simulink subsystem "phase_interpolator"  (R2022b)
settings: Solver=VariableStepAuto  StartTime=0.0  StopTime=10.0  RelTol=1e-3
undefined symbols (not defined in the file): serial_frequency, time_precision
libraries: msbPllFoundation x1, msbUtilities x1
settings Model: Creator=Ali-Laptop  LastModifiedBy=Ali-Laptop

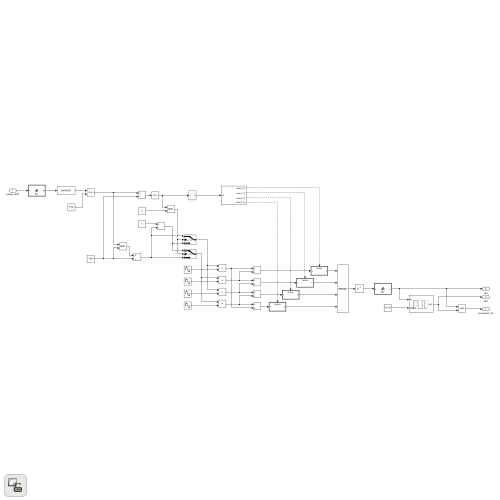
[thumbnail: Simulink's stored preview of the top-level diagram]
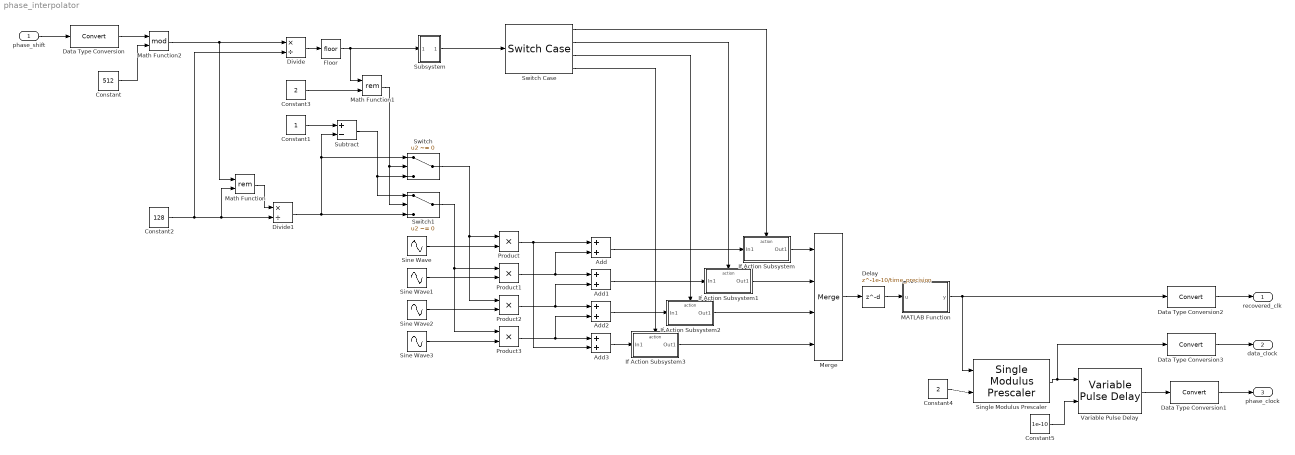
== system phase_interpolator ==
  phase_shift : Inport  SampleTime=time_precision
  Add{,1..3} (4 alike) : Sum
  Constant : Constant  Value=512
  Constant1 : Constant
  Constant2 : Constant  Value=128
  Constant3 : Constant  Value=2
  Constant4 : Constant  Value=2
  Constant5 : Constant  Value=1e-10
  Data Type Conversion{,1..3} (4 alike) : DataTypeConversion  SaturateOnIntegerOverflow=off  RndMeth=Floor
  Delay : Delay  DelayLength=1e-10/time_precision
  Divide : Product  Inputs=*/
  Divide1 : Product  Inputs=*/
  Floor : Rounding
  If Action Subsystem : Subsystem  TreatAsAtomicUnit=on
  If Action Subsystem1 : Subsystem  TreatAsAtomicUnit=on
  If Action Subsystem2 : Subsystem  TreatAsAtomicUnit=on
  If Action Subsystem3 : Subsystem  TreatAsAtomicUnit=on
  MATLAB Function : MATLAB Function  TreatAsAtomicUnit=on
  Math Function : Math  Operator=rem
  Math Function1 : Math  Operator=rem
  Math Function2 : Math  Operator=mod
  Merge : Merge  Inputs=4
  Product{,1..3} (4 alike) : Product
  Sine Wave : Sin  Frequency=pi*2*serial_frequency  SampleTime=time_precision
  Sine Wave1 : Sin  Frequency=pi*2*serial_frequency  Phase=pi/2  SampleTime=time_precision
  Sine Wave2 : Sin  Frequency=pi*2*serial_frequency  Phase=pi  SampleTime=time_precision
  Sine Wave3 : Sin  Frequency=pi*2*serial_frequency  Phase=3*pi/2  SampleTime=time_precision
  Single Modulus Prescaler : msbPllFoundation/Single Modulus Prescaler  ExtraBuffer=off  NBuffer=1
  Subsystem : Subsystem
  Subtract : Sum  Inputs=+-
  Switch : Switch  Criteria=u2 ~= 0  SaturateOnIntegerOverflow=off  InputSameDT=off
  Switch Case : SwitchCase  CaseConditions={0,1,2,3}  ShowDefaultCase=off
  Switch1 : Switch  Criteria=u2 ~= 0  SaturateOnIntegerOverflow=off  InputSameDT=off
  Variable Pulse Delay : msbUtilities/Variable Pulse Delay  InitialInput=0  BufferSize=10
  recovered_clk : Outport  SampleTime=time_precision
  data_clock : Outport  Port=2  SampleTime=time_precision
  phase_clock : Outport  Port=3  SampleTime=time_precision
  wires:
  Product/1 -> Add/1, Add3/2
  Product3/1 -> Add3/1, Add2/2
  Merge/1 -> Delay/1
  If Action Subsystem3/1(Out1) -> Merge/4
  Product1/1 -> Add/2, Add1/1
  Sine Wave3/1 -> Product3/2
  Product2/1 -> Add1/2, Add2/1
  Switch1/1 -> Product1/1, Product3/1
  Sine Wave2/1 -> Product2/2
  Constant2/1 -> Divide/2, Math Function/2, Divide1/2
  Add3/1 -> If Action Subsystem3/1(In1)
  Add/1 -> If Action Subsystem/1(In1)
  Switch/1 -> Product/1, Product2/1
  Switch Case/4 -> If Action Subsystem3/Action
  Subtract/1 -> Switch/3, Switch1/1
  Divide1/1 -> Switch1/3, Subtract/2, Switch/1
  Math Function2/1 -> Divide/1, Math Function/1
  Constant1/1 -> Subtract/1
  Math Function1/1 -> Switch/2, Switch1/2
  If Action Subsystem/1(Out1) -> Merge/1
  Divide/1 -> Floor/1
  Constant5/1 -> Variable Pulse Delay/2
  Switch Case/3 -> If Action Subsystem2/Action
  Constant3/1 -> Math Function1/2
  Sine Wave1/1 -> Product1/2
  MATLAB Function/1(y) -> Single Modulus Prescaler/1, Data Type Conversion2/1
  Add1/1 -> If Action Subsystem1/1(In1)
  If Action Subsystem1/1(Out1) -> Merge/2
  Sine Wave/1 -> Product/2
  Add2/1 -> If Action Subsystem2/1(In1)
  If Action Subsystem2/1(Out1) -> Merge/3
  Math Function/1 -> Divide1/1
  Delay/1 -> MATLAB Function/1(u)
  Constant/1 -> Math Function2/2
  Floor/1 -> Math Function1/1, Subsystem/1(In1)
  Switch Case/1 -> If Action Subsystem/Action
  Switch Case/2 -> If Action Subsystem1/Action
  Subsystem/1(Out1) -> Switch Case/1
  Data Type Conversion/1 -> Math Function2/1
  phase_shift/1 -> Data Type Conversion/1
  Data Type Conversion2/1 -> recovered_clk/1
  Constant4/1 -> Single Modulus Prescaler/2
  Single Modulus Prescaler/1 -> Variable Pulse Delay/1, Data Type Conversion3/1
  Variable Pulse Delay/1 -> Data Type Conversion1/1
  Data Type Conversion3/1 -> data_clock/1
  Data Type Conversion1/1 -> phase_clock/1

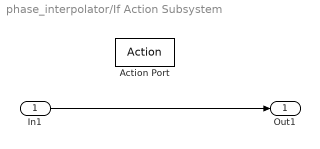
== system phase_interpolator/If Action Subsystem ==
  In1 : Inport
  Action Port : ActionPort
  Out1 : Outport  SampleTime=time_precision
  wires:
  In1/1 -> Out1/1

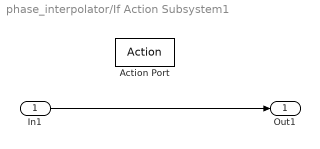
== system phase_interpolator/If Action Subsystem1 ==
  In1 : Inport
  Action Port : ActionPort
  Out1 : Outport  SampleTime=time_precision
  wires:
  In1/1 -> Out1/1

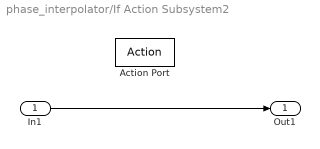
== system phase_interpolator/If Action Subsystem2 ==
  In1 : Inport
  Action Port : ActionPort
  Out1 : Outport  SampleTime=time_precision
  wires:
  In1/1 -> Out1/1

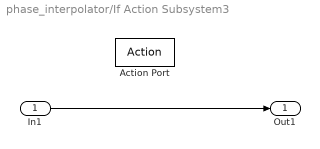
== system phase_interpolator/If Action Subsystem3 ==
  In1 : Inport
  Action Port : ActionPort
  Out1 : Outport  SampleTime=time_precision
  wires:
  In1/1 -> Out1/1

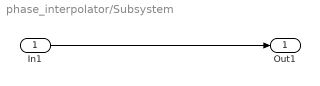
== system phase_interpolator/Subsystem ==
  In1 : Inport
  Out1 : Outport  SampleTime=time_precision
  wires:
  In1/1 -> Out1/1

== matlab function phase_interpolator/MATLAB Function ==
  data: u input; y output
function y = fcn(u)
if u > 0
    y = 1;
else
    y = 0;
end
